simulink model "vekt_shim_PMSM"  (R2019a)
settings: Solver=ode4  StartTime=0.0  StopTime=10  FixedStep=1e-5  RelTol=1e-3
libraries: simulink x6, powerlib x4, powerlib_meascontrol x1
settings Model: Creator=Sozonov_AA  LastModifiedBy=Sozonov_AA
settings DataIOCC: SaveOutput=off  SaveTime=off
settings OptimizationCC: DefaultParameterBehavior=Inlined  InlineInvariantSignals=on  EnhancedBackFolding=on  PassReuseOutputArgsAs=Individual arguments  StateBitsets=on  DataBitsets=on  ZeroExternalMemoryAtStartup=off  ZeroInternalMemoryAtStartup=off  NoFixptDivByZeroProtection=on  EfficientFloat2IntCast=on  OptimizeBlockOrder=speed  DifferentSizesBufferReuse=on
settings DebuggingCC: ParameterTunabilityLossMsg=error
settings SFSimCC: MATLABDynamicMemAlloc=off
settings RTWCC: SystemTargetFile=ert.tlc  TemplateMakefile=ert_default_tmf  GenerateReport=on  RTWVerbose=off  IncludeHyperlinkInReport=on  LaunchReport=on  GenerateTraceInfo=on  GenerateTraceReport=on  GenerateTraceReportSl=on  GenerateTraceReportSf=on  GenerateTraceReportEml=on
settings CodeAppCC: ForceParamTrailComments=on  IgnoreCustomStorageClasses=off  OperatorAnnotations=on  SimulinkDataObjDesc=on  SFDataObjDesc=on  CustomSymbolStrGlobalVar=rt$N$M  CustomSymbolStrType=$N$M  CustomSymbolStrFcn=$N$M$F  CustomSymbolStrMacro=$N$M  InsertBlockDesc=on
settings ERTTargetCC: TargetLangStandard=C99 (ISO)  GenerateSampleERTMain=on  IncludeMdlTerminateFcn=off  CombineSignalStateStructs=on  PurelyIntegerCode=on  SupportNonFinite=off  InlinedParameterPlacement=NonHierarchical  ERTCustomFileTemplate=example_file_process.tlc

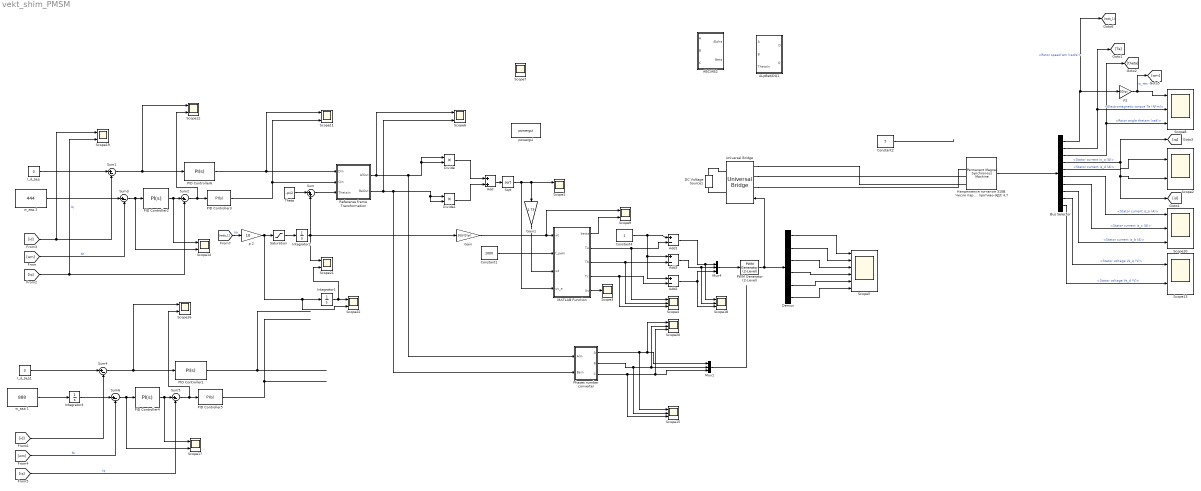
== system vekt_shim_PMSM ==
  "\tReferense frame Transformation" : Subsystem
  ABC/AB2 : Subsystem
  ALpBet\DQ1 : Subsystem
  Add : Sum
  Add1 : Sum  Inputs=+-
  Add2 : Sum  Inputs=+-
  Add3 : Sum  Inputs=+-
  Bus Selector : BusSelector  OutputSignals=Rotor speed wm (rad/s),Electromagnetic torque Te (N*m),Rotor angle thetam (rad),Stator current is_q (A),Stator current is_d (A),Stator current is_a (A),Stator current is_c (A),Stator current is_b (A),Stator voltage Vs_q (V),Stator voltage Vs_d (V)
  Constant1 : Constant  Value=1000
  Constant2 : Constant  Value=5
  Constant4 : Constant
  DC Voltage Source1 : powerlib/Electrical Sources/DC Voltage Source  Amplitude=310  Measurements=None
      settings: SourceProductName=Simscape Electrical
  Demux : Demux  Outputs=6
  Divide : Product  Inputs=**
  Divide1 : Product  Inputs=**
  Gain : Gain  Gain=360/(2*pi)
  Gain1 : Gain  Gain=1.73
  I_d_зад : Constant  Value=0
  I_d_зад1 : Constant  Value=0
  Integrator1 : Integrator  UpperSaturationLimit=2*pi  LowerSaturationLimit=0  WrappedStateUpperValue=2*pi  WrappedStateLowerValue=0  ZeroCross=off
  Integrator2 : Integrator  UpperSaturationLimit=2*pi  LowerSaturationLimit=0  WrapState=on  WrappedStateUpperValue=2*pi  WrappedStateLowerValue=0  ZeroCross=off
  Integrator3 : Integrator  LimitOutput=on  UpperSaturationLimit=444
  MATLAB Function : MATLAB Function  TreatAsAtomicUnit=on
  Mux1 : Mux  Inputs=3
  Mux4 : Mux  Inputs=3
  P2 : Gain  Gain=30/pi
  PID Controller1 : simulink/Continuous/PID Controller  Controller=PI  Form=Ideal  TimeDomain=Continuous-time  SampleTime=-1  IntegratorMethod=Forward Euler  FilterMethod=Forward Euler  ControllerParametersSource=internal  P=220/20  I=(220/20)*35  D=0  UseFilter=on  N=100  TunerSelectOption=Transfer Function Based (PID Tuner App)  InitialConditionSource=internal  InitialConditionForIntegrator=0  InitialConditionForFilter=0  DifferentiatorICPrevScaledInput=0  ExternalReset=none  TrackingMode=off  Kt=1  LimitOutput=on  UpperSaturationLimit=1000  LowerSaturationLimit=-1000  LinearizeAsGain=on  AntiWindupMode=none  Kb=1  POutMin=[]  POutMax=[]  IOutMin=[]  IOutMax=[]  DOutMin=[]  DOutMax=[]  NOutMin=[]  NOutMax=[]  SumOutMin=[]  SumOutMax=[]  SaturationOutMin=[]  SaturationOutMax=[]  PParamMin=[]  PParamMax=[]  IParamMin=[]  IParamMax=[]  DParamMin=[]  DParamMax=[]  NParamMin=[]  NParamMax=[]  KbParamMin=[]  KbParamMax=[]  KtParamMin=[]  KtParamMax=[]  KbOutMin=[]  KbOutMax=[]  KtOutMin=[]  KtOutMax=[]  IntegratorOutMin=[]  IntegratorOutMax=[]  FilterOutMin=[]  FilterOutMax=[]  SumI1OutMin=[]  SumI1OutMax=[]  SumI2OutMin=[]  SumI2OutMax=[]  SumI3OutMin=[]  SumI3OutMax=[]  SumI4OutMin=[]  SumI4OutMax=[]  SumDOutMin=[]  SumDOutMax=[]  DifferentiatorOutMin=[]  DifferentiatorOutMax=[]  FilterDiffOutCoefMin=[]  FilterDiffOutCoefMax=[]  ReciprocalOutMin=[]  ReciprocalOutMax=[]  SumDenOutMin=[]  SumDenOutMax=[]  SumNumOutMin=[]  SumNumOutMax=[]  DivideOutMin=[]  DivideOutMax=[]  IntegratorContinuousStateAttributes=''  IntegratorStateMustResolveToSignalObject=off  IntegratorRTWStateStorageClass=Auto  FilterContinuousStateAttributes=''  FilterStateMustResolveToSignalObject=off  FilterRTWStateStorageClass=Auto  ParallelPVariant=Passthrough  IdealPVariant=InternalParameters  IVariant=InternalParameters  DVariant=Disabled  IntegratorVariant=Continuous  SatVariant=Enabled  AWVariant=Passthrough  PCopyVariant=Disabled  TRVariant=Disabled  FdbkBlocksVariant=Forward  IdealPFdbkVariant=Disabled  SatFdbkVariant=Disabled  DerivativeFilterVariant=Disabled  NVariant=Disabled  NCopyVariant=Disabled_SignalSpec  FilterICVariant=Disabled  IntegratorICVariant=InternalICs  ExternalResetVariant=Disabled  TRSumVariant=Passthrough  SumFdbkVariant=Disabled  SumVariant=Sum_PI
  PID Controller2 : simulink/Continuous/PID Controller  Controller=PI  Form=Ideal  TimeDomain=Continuous-time  SampleTime=-1  IntegratorMethod=Forward Euler  FilterMethod=Forward Euler  ControllerParametersSource=internal  P=16/444  I=(16/444)*150  D=0  UseFilter=on  N=100  TunerSelectOption=Transfer Function Based (PID Tuner App)  InitialConditionSource=internal  InitialConditionForIntegrator=0  InitialConditionForFilter=0  DifferentiatorICPrevScaledInput=0  ExternalReset=none  TrackingMode=off  Kt=1  LimitOutput=on  UpperSaturationLimit=1000  LowerSaturationLimit=-1000  LinearizeAsGain=on  AntiWindupMode=none  Kb=1  POutMin=[]  POutMax=[]  IOutMin=[]  IOutMax=[]  DOutMin=[]  DOutMax=[]  NOutMin=[]  NOutMax=[]  SumOutMin=[]  SumOutMax=[]  SaturationOutMin=[]  SaturationOutMax=[]  PParamMin=[]  PParamMax=[]  IParamMin=[]  IParamMax=[]  DParamMin=[]  DParamMax=[]  NParamMin=[]  NParamMax=[]  KbParamMin=[]  KbParamMax=[]  KtParamMin=[]  KtParamMax=[]  KbOutMin=[]  KbOutMax=[]  KtOutMin=[]  KtOutMax=[]  IntegratorOutMin=[]  IntegratorOutMax=[]  FilterOutMin=[]  FilterOutMax=[]  SumI1OutMin=[]  SumI1OutMax=[]  SumI2OutMin=[]  SumI2OutMax=[]  SumI3OutMin=[]  SumI3OutMax=[]  SumI4OutMin=[]  SumI4OutMax=[]  SumDOutMin=[]  SumDOutMax=[]  DifferentiatorOutMin=[]  DifferentiatorOutMax=[]  FilterDiffOutCoefMin=[]  FilterDiffOutCoefMax=[]  ReciprocalOutMin=[]  ReciprocalOutMax=[]  SumDenOutMin=[]  SumDenOutMax=[]  SumNumOutMin=[]  SumNumOutMax=[]  DivideOutMin=[]  DivideOutMax=[]  IntegratorContinuousStateAttributes=''  IntegratorStateMustResolveToSignalObject=off  IntegratorRTWStateStorageClass=Auto  FilterContinuousStateAttributes=''  FilterStateMustResolveToSignalObject=off  FilterRTWStateStorageClass=Auto  ParallelPVariant=Passthrough  IdealPVariant=InternalParameters  IVariant=InternalParameters  DVariant=Disabled  IntegratorVariant=Continuous  SatVariant=Enabled  AWVariant=Passthrough  PCopyVariant=Disabled  TRVariant=Disabled  FdbkBlocksVariant=Forward  IdealPFdbkVariant=Disabled  SatFdbkVariant=Disabled  DerivativeFilterVariant=Disabled  NVariant=Disabled  NCopyVariant=Disabled_SignalSpec  FilterICVariant=Disabled  IntegratorICVariant=InternalICs  ExternalResetVariant=Disabled  TRSumVariant=Passthrough  SumFdbkVariant=Disabled  SumVariant=Sum_PI
  PID Controller3 : simulink/Continuous/PID Controller  Controller=PI  Form=Ideal  TimeDomain=Continuous-time  SampleTime=-1  IntegratorMethod=Forward Euler  FilterMethod=Forward Euler  ControllerParametersSource=internal  P=220/0.5  I=(220/0.5)*4  D=0  UseFilter=on  N=100  TunerSelectOption=Transfer Function Based (PID Tuner App)  InitialConditionSource=internal  InitialConditionForIntegrator=0  InitialConditionForFilter=0  DifferentiatorICPrevScaledInput=0  ExternalReset=none  TrackingMode=off  Kt=1  LimitOutput=on  UpperSaturationLimit=1000  LowerSaturationLimit=-1000  LinearizeAsGain=on  AntiWindupMode=none  Kb=1  POutMin=[]  POutMax=[]  IOutMin=[]  IOutMax=[]  DOutMin=[]  DOutMax=[]  NOutMin=[]  NOutMax=[]  SumOutMin=[]  SumOutMax=[]  SaturationOutMin=[]  SaturationOutMax=[]  PParamMin=[]  PParamMax=[]  IParamMin=[]  IParamMax=[]  DParamMin=[]  DParamMax=[]  NParamMin=[]  NParamMax=[]  KbParamMin=[]  KbParamMax=[]  KtParamMin=[]  KtParamMax=[]  KbOutMin=[]  KbOutMax=[]  KtOutMin=[]  KtOutMax=[]  IntegratorOutMin=[]  IntegratorOutMax=[]  FilterOutMin=[]  FilterOutMax=[]  SumI1OutMin=[]  SumI1OutMax=[]  SumI2OutMin=[]  SumI2OutMax=[]  SumI3OutMin=[]  SumI3OutMax=[]  SumI4OutMin=[]  SumI4OutMax=[]  SumDOutMin=[]  SumDOutMax=[]  DifferentiatorOutMin=[]  DifferentiatorOutMax=[]  FilterDiffOutCoefMin=[]  FilterDiffOutCoefMax=[]  ReciprocalOutMin=[]  ReciprocalOutMax=[]  SumDenOutMin=[]  SumDenOutMax=[]  SumNumOutMin=[]  SumNumOutMax=[]  DivideOutMin=[]  DivideOutMax=[]  IntegratorContinuousStateAttributes=''  IntegratorStateMustResolveToSignalObject=off  IntegratorRTWStateStorageClass=Auto  FilterContinuousStateAttributes=''  FilterStateMustResolveToSignalObject=off  FilterRTWStateStorageClass=Auto  ParallelPVariant=Passthrough  IdealPVariant=InternalParameters  IVariant=InternalParameters  DVariant=Disabled  IntegratorVariant=Continuous  SatVariant=Enabled  AWVariant=Passthrough  PCopyVariant=Disabled  TRVariant=Disabled  FdbkBlocksVariant=Forward  IdealPFdbkVariant=Disabled  SatFdbkVariant=Disabled  DerivativeFilterVariant=Disabled  NVariant=Disabled  NCopyVariant=Disabled_SignalSpec  FilterICVariant=Disabled  IntegratorICVariant=InternalICs  ExternalResetVariant=Disabled  TRSumVariant=Passthrough  SumFdbkVariant=Disabled  SumVariant=Sum_PI
  PID Controller4 : simulink/Continuous/PID Controller  Controller=PI  Form=Ideal  TimeDomain=Continuous-time  SampleTime=-1  IntegratorMethod=Forward Euler  FilterMethod=Forward Euler  ControllerParametersSource=internal  P=16/444  I=(16/444)*150  D=0  UseFilter=on  N=100  TunerSelectOption=Transfer Function Based (PID Tuner App)  InitialConditionSource=internal  InitialConditionForIntegrator=0  InitialConditionForFilter=0  DifferentiatorICPrevScaledInput=0  ExternalReset=none  TrackingMode=off  Kt=1  LimitOutput=on  UpperSaturationLimit=1000  LowerSaturationLimit=-1000  LinearizeAsGain=on  AntiWindupMode=none  Kb=1  POutMin=[]  POutMax=[]  IOutMin=[]  IOutMax=[]  DOutMin=[]  DOutMax=[]  NOutMin=[]  NOutMax=[]  SumOutMin=[]  SumOutMax=[]  SaturationOutMin=[]  SaturationOutMax=[]  PParamMin=[]  PParamMax=[]  IParamMin=[]  IParamMax=[]  DParamMin=[]  DParamMax=[]  NParamMin=[]  NParamMax=[]  KbParamMin=[]  KbParamMax=[]  KtParamMin=[]  KtParamMax=[]  KbOutMin=[]  KbOutMax=[]  KtOutMin=[]  KtOutMax=[]  IntegratorOutMin=[]  IntegratorOutMax=[]  FilterOutMin=[]  FilterOutMax=[]  SumI1OutMin=[]  SumI1OutMax=[]  SumI2OutMin=[]  SumI2OutMax=[]  SumI3OutMin=[]  SumI3OutMax=[]  SumI4OutMin=[]  SumI4OutMax=[]  SumDOutMin=[]  SumDOutMax=[]  DifferentiatorOutMin=[]  DifferentiatorOutMax=[]  FilterDiffOutCoefMin=[]  FilterDiffOutCoefMax=[]  ReciprocalOutMin=[]  ReciprocalOutMax=[]  SumDenOutMin=[]  SumDenOutMax=[]  SumNumOutMin=[]  SumNumOutMax=[]  DivideOutMin=[]  DivideOutMax=[]  IntegratorContinuousStateAttributes=''  IntegratorStateMustResolveToSignalObject=off  IntegratorRTWStateStorageClass=Auto  FilterContinuousStateAttributes=''  FilterStateMustResolveToSignalObject=off  FilterRTWStateStorageClass=Auto  ParallelPVariant=Passthrough  IdealPVariant=InternalParameters  IVariant=InternalParameters  DVariant=Disabled  IntegratorVariant=Continuous  SatVariant=Enabled  AWVariant=Passthrough  PCopyVariant=Disabled  TRVariant=Disabled  FdbkBlocksVariant=Forward  IdealPFdbkVariant=Disabled  SatFdbkVariant=Disabled  DerivativeFilterVariant=Disabled  NVariant=Disabled  NCopyVariant=Disabled_SignalSpec  FilterICVariant=Disabled  IntegratorICVariant=InternalICs  ExternalResetVariant=Disabled  TRSumVariant=Passthrough  SumFdbkVariant=Disabled  SumVariant=Sum_PI
  PID Controller5 : simulink/Continuous/PID Controller  Controller=PI  Form=Ideal  TimeDomain=Continuous-time  SampleTime=-1  IntegratorMethod=Forward Euler  FilterMethod=Forward Euler  ControllerParametersSource=internal  P=220/0.5  I=(220/0.5)*4  D=0  UseFilter=on  N=100  TunerSelectOption=Transfer Function Based (PID Tuner App)  InitialConditionSource=internal  InitialConditionForIntegrator=0  InitialConditionForFilter=0  DifferentiatorICPrevScaledInput=0  ExternalReset=none  TrackingMode=off  Kt=1  LimitOutput=on  UpperSaturationLimit=1000  LowerSaturationLimit=-1000  LinearizeAsGain=on  AntiWindupMode=none  Kb=1  POutMin=[]  POutMax=[]  IOutMin=[]  IOutMax=[]  DOutMin=[]  DOutMax=[]  NOutMin=[]  NOutMax=[]  SumOutMin=[]  SumOutMax=[]  SaturationOutMin=[]  SaturationOutMax=[]  PParamMin=[]  PParamMax=[]  IParamMin=[]  IParamMax=[]  DParamMin=[]  DParamMax=[]  NParamMin=[]  NParamMax=[]  KbParamMin=[]  KbParamMax=[]  KtParamMin=[]  KtParamMax=[]  KbOutMin=[]  KbOutMax=[]  KtOutMin=[]  KtOutMax=[]  IntegratorOutMin=[]  IntegratorOutMax=[]  FilterOutMin=[]  FilterOutMax=[]  SumI1OutMin=[]  SumI1OutMax=[]  SumI2OutMin=[]  SumI2OutMax=[]  SumI3OutMin=[]  SumI3OutMax=[]  SumI4OutMin=[]  SumI4OutMax=[]  SumDOutMin=[]  SumDOutMax=[]  DifferentiatorOutMin=[]  DifferentiatorOutMax=[]  FilterDiffOutCoefMin=[]  FilterDiffOutCoefMax=[]  ReciprocalOutMin=[]  ReciprocalOutMax=[]  SumDenOutMin=[]  SumDenOutMax=[]  SumNumOutMin=[]  SumNumOutMax=[]  DivideOutMin=[]  DivideOutMax=[]  IntegratorContinuousStateAttributes=''  IntegratorStateMustResolveToSignalObject=off  IntegratorRTWStateStorageClass=Auto  FilterContinuousStateAttributes=''  FilterStateMustResolveToSignalObject=off  FilterRTWStateStorageClass=Auto  ParallelPVariant=Passthrough  IdealPVariant=InternalParameters  IVariant=InternalParameters  DVariant=Disabled  IntegratorVariant=Continuous  SatVariant=Enabled  AWVariant=Passthrough  PCopyVariant=Disabled  TRVariant=Disabled  FdbkBlocksVariant=Forward  IdealPFdbkVariant=Disabled  SatFdbkVariant=Disabled  DerivativeFilterVariant=Disabled  NVariant=Disabled  NCopyVariant=Disabled_SignalSpec  FilterICVariant=Disabled  IntegratorICVariant=InternalICs  ExternalResetVariant=Disabled  TRSumVariant=Passthrough  SumFdbkVariant=Disabled  SumVariant=Sum_PI
  PID Controller6 : simulink/Continuous/PID Controller  Controller=PI  Form=Ideal  TimeDomain=Continuous-time  SampleTime=-1  IntegratorMethod=Forward Euler  FilterMethod=Forward Euler  ControllerParametersSource=internal  P=220/20  I=(220/20)*35  D=0  UseFilter=on  N=100  TunerSelectOption=Transfer Function Based (PID Tuner App)  InitialConditionSource=internal  InitialConditionForIntegrator=0  InitialConditionForFilter=0  DifferentiatorICPrevScaledInput=0  ExternalReset=none  TrackingMode=off  Kt=1  LimitOutput=on  UpperSaturationLimit=1000  LowerSaturationLimit=-1000  LinearizeAsGain=on  AntiWindupMode=none  Kb=1  POutMin=[]  POutMax=[]  IOutMin=[]  IOutMax=[]  DOutMin=[]  DOutMax=[]  NOutMin=[]  NOutMax=[]  SumOutMin=[]  SumOutMax=[]  SaturationOutMin=[]  SaturationOutMax=[]  PParamMin=[]  PParamMax=[]  IParamMin=[]  IParamMax=[]  DParamMin=[]  DParamMax=[]  NParamMin=[]  NParamMax=[]  KbParamMin=[]  KbParamMax=[]  KtParamMin=[]  KtParamMax=[]  KbOutMin=[]  KbOutMax=[]  KtOutMin=[]  KtOutMax=[]  IntegratorOutMin=[]  IntegratorOutMax=[]  FilterOutMin=[]  FilterOutMax=[]  SumI1OutMin=[]  SumI1OutMax=[]  SumI2OutMin=[]  SumI2OutMax=[]  SumI3OutMin=[]  SumI3OutMax=[]  SumI4OutMin=[]  SumI4OutMax=[]  SumDOutMin=[]  SumDOutMax=[]  DifferentiatorOutMin=[]  DifferentiatorOutMax=[]  FilterDiffOutCoefMin=[]  FilterDiffOutCoefMax=[]  ReciprocalOutMin=[]  ReciprocalOutMax=[]  SumDenOutMin=[]  SumDenOutMax=[]  SumNumOutMin=[]  SumNumOutMax=[]  DivideOutMin=[]  DivideOutMax=[]  IntegratorContinuousStateAttributes=''  IntegratorStateMustResolveToSignalObject=off  IntegratorRTWStateStorageClass=Auto  FilterContinuousStateAttributes=''  FilterStateMustResolveToSignalObject=off  FilterRTWStateStorageClass=Auto  ParallelPVariant=Passthrough  IdealPVariant=InternalParameters  IVariant=InternalParameters  DVariant=Disabled  IntegratorVariant=Continuous  SatVariant=Enabled  AWVariant=Passthrough  PCopyVariant=Disabled  TRVariant=Disabled  FdbkBlocksVariant=Forward  IdealPFdbkVariant=Disabled  SatFdbkVariant=Disabled  DerivativeFilterVariant=Disabled  NVariant=Disabled  NCopyVariant=Disabled_SignalSpec  FilterICVariant=Disabled  IntegratorICVariant=InternalICs  ExternalResetVariant=Disabled  TRSumVariant=Passthrough  SumFdbkVariant=Disabled  SumVariant=Sum_PI
  PWM Generator (2-Level) : powerlib_meascontrol/Pulse & Signal Generators/PWM Generator (2-Level)  ModulatorType=Three-phase bridge (6 pulses)  ModulatorMode=Unsynchronized  Fc=1000  Pc=90  nF=27  MinMax="[ 0  1 ]"  SamplingTechnique=Natural  ModulatingSignals=off  m=0.8  Freq=60  Phase=0  Ts=0  ShowCarrierOutport=off
  Phases number converter : Subsystem
  Saturation : Saturate  UpperLimit=inf  LowerLimit=0
  Scope{1..2,6,9,11..14,16..17,19,21..22} (13 alike) : Scope  NumInputPorts=2
  Scope{4,8,10,15,18,20} (6 alike) : Scope  NumInputPorts=3
  Scope3 : Scope
  Scope5 : Scope  NumInputPorts=6
  Scope7 : Scope
  Sqrt : Sqrt  SaturateOnIntegerOverflow=on
  Sum : Sum  Inputs=|++
  Sum{1..6} (6 alike) : Sum  Inputs=|+-
  Theta : Constant  Value=-pi/2
  Universal Bridge : powerlib/Power Electronics/Universal Bridge  Arms=3  SnubberResistance=1e5  SnubberCapacitance=inf  Device=IGBT / Diodes  Ron=1e-3  Lon=0  ForwardVoltages="[  0  0  ]"  ForwardVoltage=0  GTOparameters=[ 10e-6 , 20e-6 ]  IGBTparameters=[ 1e-6 , 2e-6 ]  Measurements=None  Measurements_2=None  converterType=Rectifier
      settings: SourceProductName=Simscape Electrical
  p 2 : Gain  Gain=10
  powergui : powerlib/powergui  Priority=1  SimulationMode=Continuous  SampleTime=50e-6  frequency=60  Iterations=50  frequencyindice=0  Pbase=100e6  ErrMax=1e-4  UnitsV=kV  UnitsW=MW  buscounter=0  FunctionMessages=off  echomessages=off  EnableUseOfTLC=off  CurrentSourceSwitches=off  DisableSnubberDevices=off  DisableRonSwitches=off  DisableVfSwitches=off  DisplayEquations=off  AutomaticDiscreteSolvers=off  SolverType=Tustin/Backward Euler (TBE)  Interpol=off  ExternalGateDelay=off  methode=off  Ts=100  x0status=blocks  SPID=on  SwTol=0  HookPort=off  NonlinearTolerance=0  nMaxIteration=15  ContinueOnMaxIteration=off  RestoreLinks=warning  ResistiveCurrentMeasurement=off  Frange=[0:2:500]  Ylog=off  Xlog=on  ShowGrid=off  save=off  variable=ZData  structure=0  ZoomFFT=off  StartTime=0.0  cycles=1  DisplayStyle=1  fundamental=60  FreqAxis=off  MaxFrequency=1000  frequencyindicesteady=1  RmsSteady=1  display=off
      settings: SourceProductName=Simscape Electrical
  w_зад 1 : Constant  Value=888
  w_зад 2 : Constant  Value=444
  "Напряжения питания 310В. Число пар полюсов 10. Момент инерции ротора 0,003 кг/м2 . Длит. момент возд. охл. 19,5 Нм. Момент трения в подшипниках 1 Нм. Зубцовый момент 1 Нм. Максимальная скорость при Ma 444 об/мин. Скорость холостого хода при Mb 533 об/мин. Длит. ток с возд. охл. 3,4 А. Ток ХХ при Mb и Nb 0,7 А. КПД при Ma и Us 84,1%. Электрическое сопротивление при 20 град. Цельсия 5,92 Ом. Индуктивность 39,8 мГн. Коэффициент момента 5,7. Коэффициент противо-ЭДС 4,7 " : powerlib/Machines/Permanent Magnet Synchronous Machine  NbPhases=3  FluxDistribution=Sinusoidal  RotorType=Round  MechanicalLoad=Torque Tm  PresetModel=No  ShowDetailedParameters=on  MeasurementBus=off  Resistance=5.92  Inductance=8.5e-3  dqInductances=[8.5e-3,8.5e-3]  La=(39.8e-3)/2  MachineConstant=Voltage Constant (V_peak L-L / krpm)  Flux=0.38  VoltageCst=689.2438  TorqueCst=5.7  Flat=120  Mechanical=[0.003 0 10 0]  PolePairs=4  InitialConditions=[0,0, 0,0]  InitialConditions5ph=[0 0 0 0 0 0]  TsPowergui=0  TsBlock=-1  RefAngle=90 degrees behind phase A axis (modified Park)
  wires:
  Gain/1 -> MATLAB Function/1(wt), Scope9/1
  MATLAB Function/1(betta) -> Scope9/2
  Constant1/1 -> MATLAB Function/2(f_pwm)
  "\tReferense frame Transformation"/1(AlOut) -> Scope6/1, Phases number converter/1(AlIn), Divide/1, Divide/2
  Add/1 -> Sqrt/1
  Divide/1 -> Add/1
  Divide1/1 -> Add/2
  Sqrt/1 -> MATLAB Function/4(us_a), Scope1/1, Gain1/1
  MATLAB Function/2(Ta) -> Add1/2, Scope4/1
  MATLAB Function/3(Tb) -> Scope4/2, Add3/2
  MATLAB Function/4(Tc) -> Scope4/3, Add2/2
  MATLAB Function/5(Us) -> Scope3/1
  Constant4/1 -> Add2/1, Add3/1, Add1/1
  Add1/1 -> Scope18/1, Mux4/1
  Add3/1 -> Mux4/2, Scope18/2
  Add2/1 -> Mux4/3, Scope18/3
  Demux/1 -> Scope5/1
  Demux/2 -> Scope5/2
  Demux/3 -> Scope5/3
  Demux/4 -> Scope5/4
  Demux/5 -> Scope5/5
  Demux/6 -> Scope5/6
  PWM Generator (2-Level)/1 -> Universal Bridge/1, Demux/1
  "Напряжения питания 310В. Число пар полюсов 10. Момент инерции ротора 0,003 кг/м2 . Длит. момент возд. охл. 19,5 Нм. Момент трения в подшипниках 1 Нм. Зубцовый момент 1 Нм. Максимальная скорость при Ma 444 об/мин. Скорость холостого хода при Mb 533 об/мин. Длит. ток с возд. охл. 3,4 А. Ток ХХ при Mb и Nb 0,7 А. КПД при Ma и Us 84,1%. Электрическое сопротивление при 20 град. Цельсия 5,92 Ом. Индуктивность 39,8 мГн. Коэффициент момента 5,7. Коэффициент противо-ЭДС 4,7 "/1 -> Bus Selector/1
  [iq] -> Scope19/2, Sum2/2  "Iq"
  Bus Selector/1 -> [rads_1], P2/1  "<Rotor speed wm (rad/s)>"
  Bus Selector/2 -> [Te], Scope8/2  "<Electromagnetic torque Te (N*m)>"
  Bus Selector/4 -> Scope2/1, [iq]  "<Stator current is_q (A)>"
  Bus Selector/5 -> [id], Scope2/2  "<Stator current is_d (A)>"
  Bus Selector/6 -> Scope10/1  "<Stator current is_a (A)>"
  Bus Selector/7 -> Scope10/2  "<Stator current is_c (A)>"
  Bus Selector/8 -> Scope10/3  "<Stator current is_b (A)>"
  Bus Selector/3 -> [theta], Scope8/3  "<Rotor angle thetam (rad)>"
  "\tReferense frame Transformation"/2(BeOut) -> Scope6/2, Phases number converter/2(Bein), Divide1/2, Divide1/1
  w_зад 2/1 -> Sum3/1
  PID Controller2/1 -> Scope14/1, Sum2/1
  Sum2/1 -> Scope12/2, PID Controller3/1
  Sum3/1 -> Scope14/2, PID Controller2/1
  Sum1/1 -> PID Controller6/1, Scope12/1
  [id] -> Scope19/1, Sum1/2
  [wm] -> Sum3/2  "Nr"
  Theta/1 -> Sum/1
  Sum/1 -> "\tReferense frame Transformation"/3(ThetaIn)
  Phases number converter/1(A) -> Scope15/1, Scope20/1, Mux1/1
  Phases number converter/2(B) -> Scope15/2, Scope20/2, Mux1/2
  Phases number converter/3(C) -> Scope15/3, Scope20/3, Mux1/3
  P2/1 -> [wm], Scope8/1  "w_тек"
  Bus Selector/9 -> Scope13/1  "<Stator voltage Vs_q (V)>"
  Bus Selector/10 -> Scope13/2  "<Stator voltage Vs_d (V)>"
  Mux4/1 -> PWM Generator (2-Level)/1
  Gain1/1 -> MATLAB Function/3(ud)
  Mux1/1 -> ?
  [wm] -> Sum6/2  "Nr"
  [id] -> Sum4/2
  Sum4/1 -> PID Controller1/1, Scope16/1
  Sum6/1 -> PID Controller4/1, Scope17/2
  PID Controller1/1 -> ?
  Sum5/1 -> PID Controller5/1, Scope16/2
  I_d_зад1/1 -> Sum4/1
  PID Controller4/1 -> Sum5/1, Scope17/1
  Integrator3/1 -> Sum6/1
  PID Controller5/1 -> ?
  w_зад 1/1 -> Integrator3/1
  [iq] -> Sum5/2  "Iq"
  PID Controller6/1 -> "\tReferense frame Transformation"/1(Din), Scope11/1
  PID Controller3/1 -> "\tReferense frame Transformation"/2(Qin), Scope11/2
  I_d_зад/1 -> Sum1/1
  Constant2/1 -> ?
  [rads_1] -> p 2/1  "Nr"
  Integrator2/1 -> Scope21/1, Gain/1, Sum/2
  Integrator1/1 -> Scope21/2, Scope22/1
  p 2/1 -> Saturation/1, Scope22/2, Integrator1/1
  Saturation/1 -> Integrator2/1
  connections:
  Universal Bridge/LConn1 -- "Напряжения питания 310В. Число пар полюсов 10. Момент инерции ротора 0,003 кг/м2 . Длит. момент возд. охл. 19,5 Нм. Момент трения в подшипниках 1 Нм. Зубцовый момент 1 Нм. Максимальная скорость при Ma 444 об/мин. Скорость холостого хода при Mb 533 об/мин. Длит. ток с возд. охл. 3,4 А. Ток ХХ при Mb и Nb 0,7 А. КПД при Ma и Us 84,1%. Электрическое сопротивление при 20 град. Цельсия 5,92 Ом. Индуктивность 39,8 мГн. Коэффициент момента 5,7. Коэффициент противо-ЭДС 4,7 "/LConn1
  Universal Bridge/LConn3 -- "Напряжения питания 310В. Число пар полюсов 10. Момент инерции ротора 0,003 кг/м2 . Длит. момент возд. охл. 19,5 Нм. Момент трения в подшипниках 1 Нм. Зубцовый момент 1 Нм. Максимальная скорость при Ma 444 об/мин. Скорость холостого хода при Mb 533 об/мин. Длит. ток с возд. охл. 3,4 А. Ток ХХ при Mb и Nb 0,7 А. КПД при Ma и Us 84,1%. Электрическое сопротивление при 20 град. Цельсия 5,92 Ом. Индуктивность 39,8 мГн. Коэффициент момента 5,7. Коэффициент противо-ЭДС 4,7 "/LConn3
  Universal Bridge/LConn2 -- "Напряжения питания 310В. Число пар полюсов 10. Момент инерции ротора 0,003 кг/м2 . Длит. момент возд. охл. 19,5 Нм. Момент трения в подшипниках 1 Нм. Зубцовый момент 1 Нм. Максимальная скорость при Ma 444 об/мин. Скорость холостого хода при Mb 533 об/мин. Длит. ток с возд. охл. 3,4 А. Ток ХХ при Mb и Nb 0,7 А. КПД при Ma и Us 84,1%. Электрическое сопротивление при 20 град. Цельсия 5,92 Ом. Индуктивность 39,8 мГн. Коэффициент момента 5,7. Коэффициент противо-ЭДС 4,7 "/LConn2
  DC Voltage Source1/RConn1 -- Universal Bridge/RConn1
  DC Voltage Source1/LConn1 -- Universal Bridge/RConn2

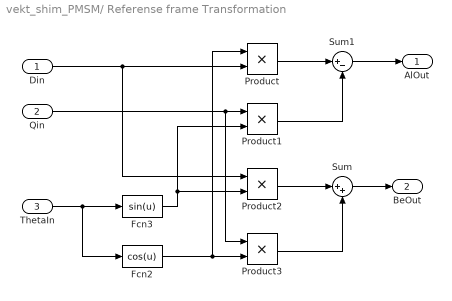
== system vekt_shim_PMSM/	Referense frame Transformation ==
  Din : Inport
  Qin : Inport  Port=2
  ThetaIn : Inport  Port=3
  Fcn2 : Fcn  Expr=cos(u)
  Fcn3 : Fcn  Expr=sin(u)
  Product{,1..3} (4 alike) : Product  RndMeth=Zero
  Sum : Sum  Inputs=|++
  Sum1 : Sum  Inputs=|+-
  AlOut : Outport
  BeOut : Outport  Port=2
  wires:
  ThetaIn/1 -> Fcn2/1, Fcn3/1
  Product/1 -> Sum1/1
  Product1/1 -> Sum1/2
  Sum1/1 -> AlOut/1
  Sum/1 -> BeOut/1
  Product2/1 -> Sum/1
  Product3/1 -> Sum/2
  Fcn2/1 -> Product/1, Product3/2
  Din/1 -> Product/2, Product2/1
  Qin/1 -> Product3/1, Product1/1
  Fcn3/1 -> Product1/2, Product2/2

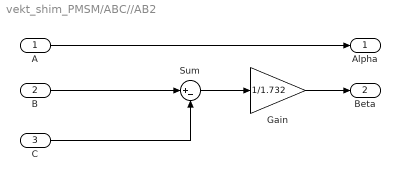
== system vekt_shim_PMSM/ABC//AB2 ==
  A : Inport
  B : Inport  Port=2
  C : Inport  Port=3
  Gain : Gain  Gain=1/1.732
  Sum : Sum  Inputs=|+-
  Alpha : Outport
  Beta : Outport  Port=2
  wires:
  Gain/1 -> Beta/1
  A/1 -> Alpha/1
  Sum/1 -> Gain/1
  C/1 -> Sum/2
  B/1 -> Sum/1

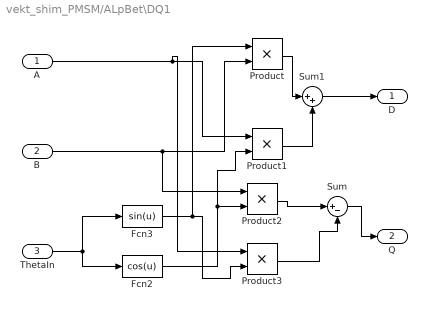
== system vekt_shim_PMSM/ALpBet\DQ1 ==
  A : Inport
  B : Inport  Port=2
  ThetaIn : Inport  Port=3
  Fcn2 : Fcn  Expr=cos(u)
  Fcn3 : Fcn  Expr=sin(u)
  Product{,1..3} (4 alike) : Product  RndMeth=Zero
  Sum : Sum  Inputs=|+-
  Sum1 : Sum  Inputs=|++
  D : Outport
  Q : Outport  Port=2
  wires:
  Product3/1 -> Sum/2
  Product2/1 -> Sum/1
  Sum/1 -> Q/1
  Sum1/1 -> D/1
  Product1/1 -> Sum1/2
  Product/1 -> Sum1/1
  A/1 -> Product3/1, Product1/1
  Fcn2/1 -> Product2/2, Product1/2
  Fcn3/1 -> Product3/2, Product/1
  B/1 -> Product2/1, Product/2
  ThetaIn/1 -> Fcn2/1, Fcn3/1

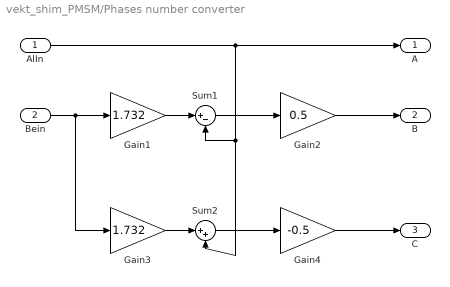
== system vekt_shim_PMSM/Phases number converter ==
  AlIn : Inport
  Bein : Inport  Port=2
  Gain1 : Gain  Gain=1.732
  Gain2 : Gain  Gain=0.5
  Gain3 : Gain  Gain=1.732
  Gain4 : Gain  Gain=-0.5
  Sum1 : Sum  Inputs=|+-
  Sum2 : Sum  Inputs=|++
  A : Outport
  B : Outport  Port=2
  C : Outport  Port=3
  wires:
  AlIn/1 -> A/1, Sum1/2, Sum2/2
  Bein/1 -> Gain1/1, Gain3/1
  Gain1/1 -> Sum1/1
  Sum1/1 -> Gain2/1
  Gain2/1 -> B/1
  Gain3/1 -> Sum2/1
  Sum2/1 -> Gain4/1
  Gain4/1 -> C/1

== matlab function vekt_shim_PMSM/MATLAB Function ==
  data: wt input; betta output double; f_pwm input; ud input; us_a input; Ta output double; Tb output double; Tc output double; Us output double
function [ betta, Ta, Tb, Tc, Us] = fcn(wt, f_pwm, ud, us_a)

v=0;
t_pwm = (1/f_pwm);
Us = sqrt(3)*us_a/ud;


if (wt >= 0 && wt < 60)%базовый вектор 1
    v=1;
end    
if (wt > 60 && wt < 120)%базовый вектор 2
    v=2;
end
if (wt > 120 && wt < 180)%базовый вектор 3
    v=3;  
end
if (wt > 180 && wt < 240)%базовый вектор 4
    v=4; 
end
if (wt > 240 && wt < 300)%базовый вектор 5
    v=5; 
end
if (wt > 300 && wt <= 360)%базовый вектор 6
    v=6;      
end
   
betta=60-(v*60-wt);

T_1=Us*sin((60-betta)*2*pi/360);
T_2=Us*sin((betta)*2*pi/360);
T_0=1-T_1-T_2;

t_1=T_1+T_2+(T_0/2);
t_2=T_2+(T_0/2);
t_3=T_1+(T_0/2);
Ta=0;
Tb=0;
Tc=0;

if(v==1)
    Ta=t_1;
    Tb=t_2;
    Tc=T_0/2;
end    
if(v==2)
    Ta=t_3;
    Tb=t_1;
    Tc=T_0/2;
end
if(v==3)
    Ta=T_0/2;
    Tb=t_1;
    Tc=t_2;
end
if(v==4)
    Ta=T_0/2;
    Tb=t_3;
    Tc=t_1;
end
if(v==5)
    Ta=t_2;
    Tb=T_0/2;
    Tc=t_1;
end
if(v==6)
    Ta=t_1;
    Tb=T_0/2;
    Tc=t_3;
end
